simulink model "innerflow"  (Simulink 6.4)
settings: Solver=ode45  StartTime=0.0  StopTime=inf  RelTol=1e-3
settings Model: LastModifiedBy=rsnah

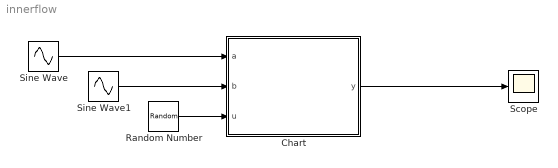
== system innerflow ==
  Chart : Stateflow chart
  Random Number : RandomNumber  SampleTime=0
  Scope : Scope
  Sine Wave : Sin  SampleTime=0
  Sine Wave1 : Sin  Frequency=1.5  Phase=-1  SampleTime=0
  wires:
  Chart/1(y) -> Scope/1
  Sine Wave/1 -> Chart/1(a)
  Sine Wave1/1 -> Chart/2(b)
  Random Number/1 -> Chart/3(u)

== stateflow chart Chart ==
  state A
    (default) -> (junction 5)
    (junction 5) -> (junction 6) [order 2] : {
        | y = -1;
        | }
    (junction 5) -> (junction 7) [order 1] : [a > 0]
    (junction 7) -> (junction 8) : {
        | y = 1;
        | }
    (junction 8) -> (junction 6)
  state B
    (default) -> (junction 9)
    (junction 9) -> (junction 10) [order 1] : [a > 0]
    (junction 9) -> (junction 11) [order 2] : {
        | y = 0;
        | }
    (junction 10) -> (junction 12) : {
        | y = u;
        | }
    (junction 12) -> (junction 11)
    B -> (junction 9) [order 1]
  (default) -> A
  A -> B : [b > 0]
  B -> A [order 1] : [b < 0]
  data: a input inherited; b input inherited; u input inherited; y output double =0
